simulink model "Identification_rotationalVel"  (R2020a)
settings: Solver=VariableStepAuto  StartTime=0.0  StopTime=10.0  RelTol=1e-3
values from neighbouring files (symbols this model uses):
  Kphi = 0.0075    [OuterLoop_rotVel_phi.m]    (also in Part3_Identification_rotVel.m; Part4_InnerLoop_rotVel.m)
  rotationalVelocity = 1.50    (= 1.5)    [Part3_Identification_rotVel.m]
  sigphi = 20    [OuterLoop_rotVel_phi.m]    (also in Part3_Identification_rotVel.m = 10; Part4_InnerLoop_rotVel.m)
  Vin = 200    [Part3_Identification_forVel.m]    (also in Part3_Identification_rotVel.m)
settings Model: Creator=brett  LastModifiedBy=brett

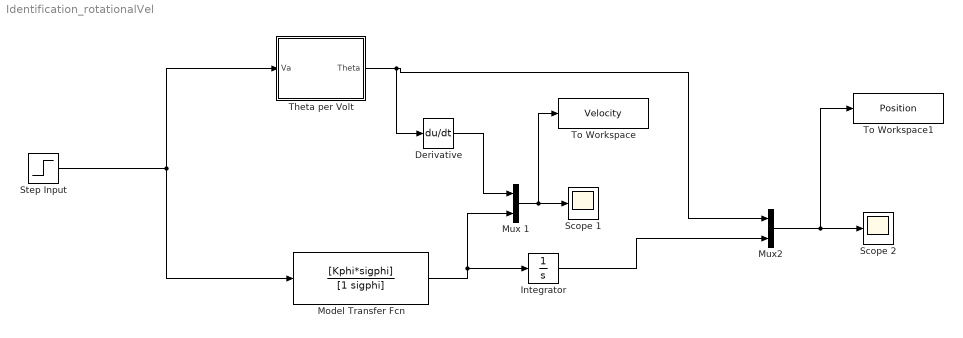
== system Identification_rotationalVel ==
  Derivative : Derivative
  Integrator : Integrator
  Model Transfer Fcn : TransferFcn  Numerator=[Kphi*sigphi]  Denominator=[1 sigphi]
  Mux 1 : Mux  Inputs=2
  Mux2 : Mux  Inputs=2
  Scope 1 : Scope
  Scope 2 : Scope
  Step Input : Step  After=200  SampleTime=0
  Theta per Volt : Subsystem
  To Workspace : ToWorkspace  VariableName=Velocity  SaveFormat=Timeseries  SampleTime=-1
  To Workspace1 : ToWorkspace  VariableName=Position  SaveFormat=Timeseries  SampleTime=-1
  wires:
  Step Input/1 -> Model Transfer Fcn/1, Theta per Volt/1(Va)
  Model Transfer Fcn/1 -> Mux 1/2, Integrator/1
  Derivative/1 -> Mux 1/1
  Integrator/1 -> Mux2/2
  Theta per Volt/1(Theta) -> Derivative/1, Mux2/1
  Mux2/1 -> To Workspace1/1, Scope 2/1
  Mux 1/1 -> To Workspace/1, Scope 1/1

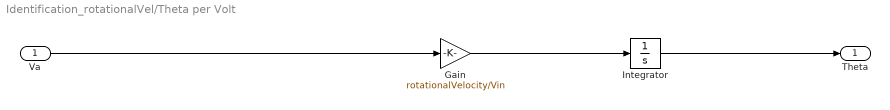
== system Identification_rotationalVel/Theta per Volt ==
  Va : Inport
  Gain : Gain  Gain=rotationalVelocity/Vin
  Integrator : Integrator
  Theta : Outport
  wires:
  Va/1 -> Gain/1
  Gain/1 -> Integrator/1
  Integrator/1 -> Theta/1
